simulink model "LOSR_old"  (R2022a)
settings: Solver=FixedStepDiscrete  StartTime=0.0  StopTime=0.04  FixedStep=0.04  RelTol=1e-3
PreLoadFcn:
  | listing = dir;
  | if (contains([listing .name], 'AGR')) && (contains([listing .name], 'MAP'))
  |     addpath('./AGR', './MAP');
  |     addpath( genpath('./MAP') );
  | elseif (contains([listing .name], 'LOSR.slx'))
  |     addpath('../AGR', '../MAP');
  |     addpath( genpath('../MAP') );
  | else
  | 
  | end
  | 
  | load('BusStructureLOSR.mat');
InitFcn:
  | listing = dir;
  | if (contains([listing .name], 'AGR')) && (contains([listing .name], 'MAP'))
  |     addpath('./AGR', './MAP');
  |     addpath( genpath('./MAP') );
  | elseif (contains([listing .name], 'LOSR.slx'))
  |     addpath('../AGR', '../MAP');
  |     addpath( genpath('../MAP') );
  | else
  | 
  | end
  | 
  | load('BusStructureLOSR.mat');
StartFcn:
  | listing = dir;
  | if (contains([listing .name], 'AGR')) && (contains([listing .name], 'MAP'))
  |     addpath('./AGR', './MAP');
  |     addpath( genpath('./MAP') );
  | elseif (contains([listing .name], 'LOSR.slx'))
  |     addpath('../AGR', '../MAP');
  |     addpath( genpath('../MAP') );
  | else
  | 
  | end
  | 
  | load('BusStructureLOSR.mat');
undefined symbols (not defined in the file): b2NED, delLLH, heading, llh, losECEF, losGeod, LOSRDataTagWrap, LOSRDataValid, LOSRDirectionCosineX, LOSRDirectionCosineY, LOSRDirectionCosineZ, LOSRSelected, LOSRSelectedWraparound, LOSRTargetElevation, LOSRTargetLatitude, LOSRTargetLongitude, LOSRTargetRangeEast, LOSRTargetRangeNorth, LOSRTargetRangeVertical, ne, ned2ECEF, pECEF_ref, pitch, roll, testLLH, testLLH2, testTerrainHeight
settings Model: Creator=ASCL  LastModifiedBy=ASCL
settings SolverCC: AlgebraicLoopSolver=TrustRegion
settings DataIOCC: SaveOutput=off  SignalLogging=off  DSMLogging=off  SaveTime=off  ReturnWorkspaceOutputs=off
settings OptimizationCC: DefaultParameterBehavior=Inlined  UseDivisionForNetSlopeComputation=on  GainParamInheritBuiltInType=on  UseFloatMulNetSlope=on  InlineInvariantSignals=on  BufferReuse=off  ExpressionFolding=off  PassReuseOutputArgsAs=Individual arguments  ZeroExternalMemoryAtStartup=off  ZeroInternalMemoryAtStartup=off  EfficientMapNaN2IntZero=off  LifeSpan=1  OptimizeBlockOrder=speed  DifferentSizesBufferReuse=on  EfficientTunableParamExpr=on
settings DebuggingCC: ParameterTunabilityLossMsg=error  UnconnectedInputMsg=warning  UnconnectedOutputMsg=warning  UnconnectedLineMsg=warning  SFMachineParentedDataDiag=warning  ArithmeticOperatorsInVariantConditions=warning
settings HardwareCC: ProdBitPerPointer=32  ProdBitPerSizeT=32  ProdBitPerPtrDiffT=32  ProdLargestAtomicInteger=Long  ProdLargestAtomicFloat=Double  ProdEndianess=BigEndian  ProdWordSize=32  ProdLongLongMode=on  ProdHWDeviceType=Freescale->MPC83xx
settings ModelReferenceCC: ModelReferenceNumInstancesAllowed=Single
settings SFSimCC: SimUserLibraries=MAPd.lib WS2_32.lib  SimUseLocalCustomCode=off  MATLABDynamicMemAlloc=off  CustomCodeUndefinedFunction=UseInterfaceOnly
settings SFSimCC: SimCustomHeaderCode=|
  | #include "MAP.h"
  | #include "DVOF.h"
  | #include "MAPDATA.h"
  | #include "userDefined.h"
settings SFSimCC: SimUserSources=|
  | MAP.c
  | DVOF.c
  | userDefined.c
settings RTWCC: SystemTargetFile=ert.tlc  TemplateMakefile=ert_default_tmf  GenerateReport=on  RTWUseLocalCustomCode=off  RTWUseSimCustomCode=on  CustomLibrary=MAPd.lib WS2_32.lib  IncludeHyperlinkInReport=on  LaunchReport=on  GenerateTraceInfo=on  GenerateTraceReport=on  GenerateTraceReportSl=on  GenerateTraceReportSf=on  GenerateTraceReportEml=on  GenerateCodeMetricsReport=on
settings RTWCC: CustomHeaderCode=|
  | #include "MAP.h"
  | #include "DVOF.h"
  | #include "MAPDATA.h"
  | #include "userDefined.h"
settings RTWCC: CustomSource=|
  | MAP.c
  | DVOF.c
  | userDefined.c
settings CodeAppCC: ForceParamTrailComments=on  IgnoreCustomStorageClasses=off  OperatorAnnotations=on  SimulinkDataObjDesc=on  SFDataObjDesc=on  InsertBlockDesc=on  EnableCustomComments=on
settings ERTTargetCC: TargetLangStandard=C99 (ISO)  UtilityFuncGeneration=Shared location  GenerateSampleERTMain=on  IncludeMdlTerminateFcn=off  CombineSignalStateStructs=on  SuppressErrorStatus=on  SupportAbsoluteTime=off  SupportComplex=off  InlinedParameterPlacement=NonHierarchical  ERTCustomFileTemplate=example_file_process.tlc  ERTFilePackagingFormat=CompactWithDataFile  EnableSignedLeftShifts=off  EnableSignedRightShifts=off

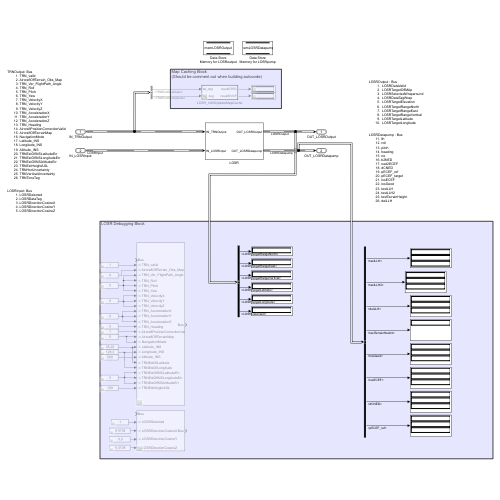
[thumbnail: Simulink's stored preview of the top-level diagram]
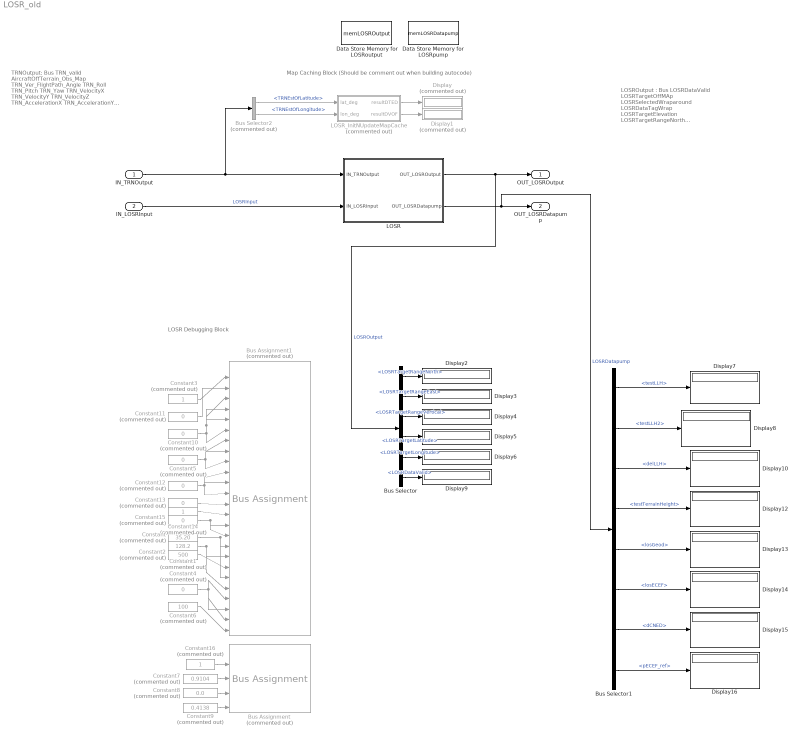
== system LOSR_old ==
  note: LOSR Debugging Block
  note: TRNOutput: Bus
      | TRN_valid
      | AircraftOffTerrain_Obs_Map
      | TRN_Ver_FlightPath_Angle
      | TRN_Roll
      | TRN_Pitch
      | TRN_Yaw
      | TRN_VelocityX
      | TRN_VelocityY
      | TRN_VelocityZ
      | TRN_AccelerationX
      | TRN_AccelerationY
      | TRN_AccelerationZ
      | TRN_Heading
      | AircraftPositionCorrectionValid
      | AircraftOffTerrainMap
      | NavigationMode
      | Latitude_INS
      | Longitude_INS
      | Altitude_INS
      | TRNEstOfINSLatitudeErr
      | TRNEstOfINSLongitudeErr
      | TRNEstOfINSAltitudeErr
      | TRNEstHeightAGL
      | TRNHorUncertainty
      | TRNVerticalUncertainty
      | TRNTimeTag
      |
      | LOSRInput: Bus
      | LOSRSelected
      | LOSRDataTag
      | LOSRDirectionCosineX
      | LOSRDirectionCosineY
      | LOSRDirectionCosineZ
  note: LOSROutput : Bus
      | LOSRDataValid
      | LOSRTargetOffMAp
      | LOSRSelectedWraparound
      | LOSRDataTagWrap
      | LOSRTargetElevation
      | LOSRTargetRangeNorth
      | LOSRTargetRangeEast
      | LOSRTargetRangeVertical
      | LOSRTargetLatitude
      | LOSRTargetLongitude
      |
      | LOSRDatapump : Bus
      | 11. llh
      | 12. roll
      | 13. pitch
      | 14. heading
      | 15. ne
      | 16. b2NED
      | 17. ned2ECEF
      | 18. dCNED
      | 19. pECEF_ref
      | 20. pECEF_target
      | 21. losECEF
      | 22. losGeod
      | 23. testLLH
      | 24. testLLH2
      | 25. testTerrainHeight
      | 26. delLLH
  note: Map Caching Block
      | (Should be comment out when building autocode)
  IN_TRNOutput : Inport  OutDataTypeStr=Bus: TRNOutput  BusOutputAsStruct=on
  IN_LOSRInput : Inport  Port=2  OutDataTypeStr=Bus: LOSRInput  BusOutputAsStruct=on
  Bus Assignment : BusAssignment  Commented=on  AssignedSignals=LOSRSelected,LOSRDirectionCosineX,LOSRDirectionCosineY,LOSRDirectionCosineZ
  Bus Assignment1 : BusAssignment  Commented=on  AssignedSignals=TRN_valid,AircraftOffTerrain_Obs_Map,TRN_Ver_FlightPath_Angle,TRN_Roll,TRN_Pitch,TRN_Yaw,TRN_VelocityX,TRN_VelocityY,TRN_VelocityZ,TRN_AccelerationX,TRN_AccelerationY,TRN_AccelerationZ,TRN_Heading,AircraftPositionCorrectionValid,AircraftOffTerrainMap,NavigationMode,Latitude_INS,Longitude_INS,Altitude_INS,TRNEstOfLatitude,TRNEstOfLongitude,TRNEstOfINSLatitudeErr,TRNEstOfINSLongitudeErr,TRNEstOfINSAltitudeErr,TRNEstHeightAGL
  Bus Selector : BusSelector  OutputSignals=LOSRTargetRangeNorth,LOSRTargetRangeEast,LOSRTargetRangeVertical,LOSRTargetLatitude,LOSRTargetLongitude,LOSRDataValid
  Bus Selector1 : BusSelector  OutputSignals=testLLH,testLLH2,delLLH,testTerrainHeight,losGeod,losECEF,dCNED,pECEF_ref
  Bus Selector2 : BusSelector  Commented=on  OutputSignals=TRNEstOfLatitude,TRNEstOfLongitude
  Constant : Constant  Commented=on  Value=35.20
  Constant1 : Constant  Commented=on  Value=128.2
  Constant{4..5,10,12..13} (5 alike) : Constant  Commented=on  Value=0
  Constant11 : Constant  Commented=on  Value=0  OutDataTypeStr=boolean
  Constant14 : Constant  Commented=on  OutDataTypeStr=boolean
  Constant15 : Constant  Commented=on  Value=0  OutDataTypeStr=boolean
  Constant16 : Constant  Commented=on  OutDataTypeStr=boolean
  Constant2 : Constant  Commented=on  Value=500
  Constant3 : Constant  Commented=on  OutDataTypeStr=boolean
  Constant6 : Constant  Commented=on  Value=100  OutDataTypeStr=uint16
  Constant7 : Constant  Commented=on  Value=0.9104
  Constant8 : Constant  Commented=on  Value=0.0
  Constant9 : Constant  Commented=on  Value=0.4138
  Data Store Memory for LOSRoutput : DataStoreMemory  DataStoreName=memLOSROutput  ReadBeforeWriteMsg=warning  WriteAfterWriteMsg=warning  WriteAfterReadMsg=warning  VectorParams1D=off  ShowAdditionalParam=off  OutDataTypeStr=Bus: LOSROutput
  Data Store Memory for LOSRpump : DataStoreMemory  DataStoreName=memLOSRDatapump  ReadBeforeWriteMsg=warning  WriteAfterWriteMsg=warning  WriteAfterReadMsg=warning  VectorParams1D=off  ShowAdditionalParam=off  OutDataTypeStr=Bus: LOSRDatapump
  Display : Display  Commented=on
  Display1 : Display  Commented=on
  Display{2..10,12..16} (14 alike) : Display
  LOSR : Subsystem
      mask init:
      | % latGPS = double(0);
      | % lonGPS = double(0);
      | % altGPS = double(0);
      | % velEGPS = double(0);
      | % velNGPS = double(0);
      | % velUGPS = double(0);
      | % notValidGPS = boolean(0);
      | % notAvaildINS = boolean(0);
      | % velUINS = double(0);
      | % velVINS = double(0);
      | % velWINS = double(0);
      | % rollINS = double(0);
      | % pitchINS = double(0);
      | % hgdINS = double(0);
      | % accXINS = double(0);
      | % accYINS = double(0);
      | % accZINS = double(0);
      | % activated = boolean(0);
      | % reactionT = uint16(0);
      | % pullUpG = uint16(0);
      | % rollRate = uint16(0);
      | % gOnsetRate = uint16(0);
      | % maxGamma = uint16(0);
      | % setWarnH = double(0);
      | % obsWarningTime = uint16(1);
      | % wiresWarningTime = uint16(1);
      | % latErrOfINS = double(0);
      | % lonErrOfINS = double(0);
      | % altErrorofINS = uint16(0);
      | % heightEstOfTRN = uint16(0);
      | % horUncertaintyOfTRN = double(0);
      | % verUncertaintyOfTRN = double(0);
  LOSR_InitNUpdateMapCache : Subsystem  Commented=on  TreatAsAtomicUnit=on
  OUT_LOSROutput : Outport  OutDataTypeStr=Bus: LOSROutput  VectorParamsAs1DForOutWhenUnconnected=off  BusOutputAsStruct=on
  OUT_LOSRDatapump : Outport  Port=2  OutDataTypeStr=Bus: LOSRDatapump  VectorParamsAs1DForOutWhenUnconnected=off  BusOutputAsStruct=on
  wires:
  LOSR/2(OUT_LOSRDatapump) -> Bus Selector1/1, OUT_LOSRDatapump/1  "LOSRDatapump"
  LOSR/1(OUT_LOSROutput) -> Bus Selector/1, OUT_LOSROutput/1  "LOSROutput"
  LOSR_InitNUpdateMapCache/2(resultDVOF) -> Display1/1
  Bus Selector/1 -> Display2/1  "<LOSRTargetRangeNorth>"
  Bus Selector/5 -> Display6/1  "<LOSRTargetLongitude>"
  Bus Selector/4 -> Display5/1  "<LOSRTargetLatitude>"
  Bus Selector/3 -> Display4/1  "<LOSRTargetRangeVertical>"
  Bus Selector/2 -> Display3/1  "<LOSRTargetRangeEast>"
  Bus Selector1/1 -> Display7/1  "<testLLH>"
  Bus Selector1/2 -> Display8/1  "<testLLH2>"
  Bus Selector/6 -> Display9/1  "<LOSRDataValid>"
  Bus Selector1/3 -> Display10/1  "<delLLH>"
  Bus Selector1/4 -> Display12/1  "<testTerrainHeight>"
  Bus Selector1/5 -> Display13/1  "<losGeod>"
  Bus Selector1/6 -> Display14/1  "<losECEF>"
  Bus Selector1/7 -> Display15/1  "<dCNED>"
  Bus Selector1/8 -> Display16/1  "<pECEF_ref>"
  LOSR_InitNUpdateMapCache/1(resultDTED) -> Display/1
  Constant9/1 -> Bus Assignment/5
  Constant7/1 -> Bus Assignment/3
  Constant8/1 -> Bus Assignment/4
  Constant1/1 -> Bus Assignment1/22, Bus Assignment1/19
  Constant/1 -> Bus Assignment1/21, Bus Assignment1/18
  Constant2/1 -> Bus Assignment1/20
  Constant4/1 -> Bus Assignment1/23, Bus Assignment1/25, Bus Assignment1/24
  Constant5/1 -> Bus Assignment1/10, Bus Assignment1/8, Bus Assignment1/9
  Constant10/1 -> Bus Assignment1/7, Bus Assignment1/4, Bus Assignment1/5, Bus Assignment1/6
  Constant3/1 -> Bus Assignment1/2
  Constant11/1 -> Bus Assignment1/3
  Constant12/1 -> Bus Assignment1/13, Bus Assignment1/11, Bus Assignment1/12
  Constant13/1 -> Bus Assignment1/14
  Constant14/1 -> Bus Assignment1/15
  Constant15/1 -> Bus Assignment1/17, Bus Assignment1/16
  Constant6/1 -> Bus Assignment1/26
  Bus Selector2/1 -> LOSR_InitNUpdateMapCache/1(lat_deg)  "<TRNEstOfLatitude>"
  Bus Selector2/2 -> LOSR_InitNUpdateMapCache/2(lon_deg)  "<TRNEstOfLongitude>"
  Constant16/1 -> Bus Assignment/2
  IN_TRNOutput/1 -> Bus Selector2/1, LOSR/1(IN_TRNOutput)
  IN_LOSRInput/1 -> LOSR/2(IN_LOSRInput)  "LOSRInput"

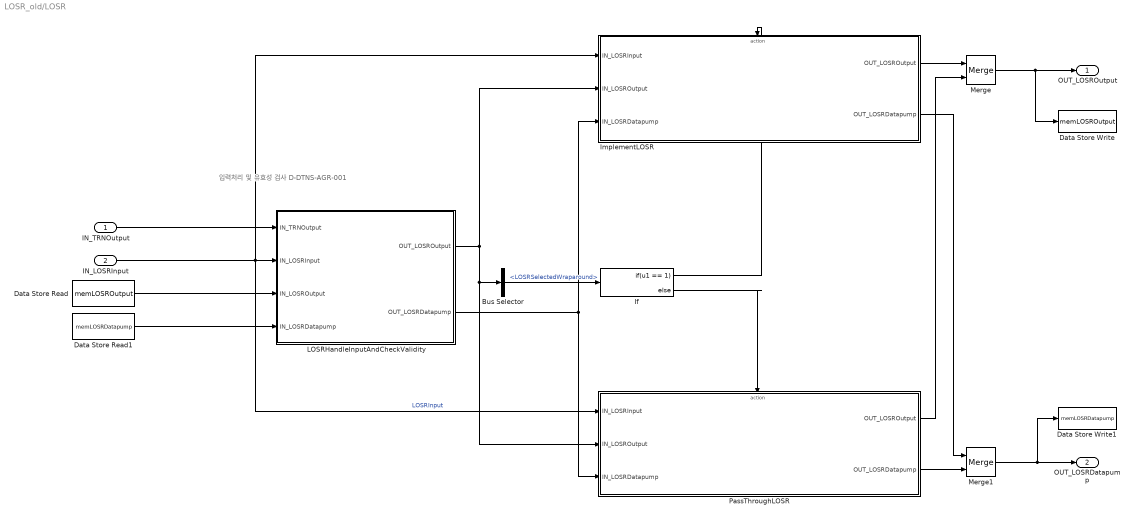
== system LOSR_old/LOSR ==
  note: 입력처리 및 유효성 검사 D-DTNS-AGR-001
  IN_TRNOutput : Inport  OutDataTypeStr=Bus: TRNOutput
  IN_LOSRInput : Inport  Port=2  OutDataTypeStr=Bus: LOSRInput
  Bus Selector : BusSelector  OutputSignals=LOSRSelectedWraparound
  Data Store Read : DataStoreRead  DataStoreName=memLOSROutput  IndexOptions=Index vector (dialog)  Indices=1  OutputSizes=1
  Data Store Read1 : DataStoreRead  DataStoreName=memLOSRDatapump  IndexOptions=Index vector (dialog)  Indices=1  OutputSizes=1
  Data Store Write : DataStoreWrite  DataStoreName=memLOSROutput  IndexOptions=Index vector (dialog)  Indices=1  OutputSizes=1
  Data Store Write1 : DataStoreWrite  DataStoreName=memLOSRDatapump  IndexOptions=Index vector (dialog)  Indices=1  OutputSizes=1
  If : If  IfExpression=u1 == 1
  ImplementLOSR : Subsystem  TreatAsAtomicUnit=on
      settings: RTWSystemCode=Nonreusable function  RTWFcnNameOpts=Use subsystem name
  LOSRHandleInputAndCheckValidity : Subsystem  TreatAsAtomicUnit=on
      settings: RTWSystemCode=Nonreusable function  RTWFcnNameOpts=Use subsystem name
  Merge : Merge
  Merge1 : Merge
  PassThroughLOSR : Subsystem  TreatAsAtomicUnit=on
      settings: RTWSystemCode=Nonreusable function  RTWFcnNameOpts=Use subsystem name
  OUT_LOSROutput : Outport  OutDataTypeStr=Bus: LOSROutput  VectorParamsAs1DForOutWhenUnconnected=off
  OUT_LOSRDatapump : Outport  Port=2  OutDataTypeStr=Bus: LOSRDatapump  VectorParamsAs1DForOutWhenUnconnected=off
  wires:
  IN_LOSRInput/1 -> ImplementLOSR/1(IN_LOSRInput), PassThroughLOSR/1(IN_LOSRInput), LOSRHandleInputAndCheckValidity/2(IN_LOSRInput)  "LOSRInput"
  LOSRHandleInputAndCheckValidity/1(OUT_LOSROutput) -> ImplementLOSR/2(IN_LOSROutput), Bus Selector/1, PassThroughLOSR/2(IN_LOSROutput)
  Bus Selector/1 -> If/1  "<LOSRSelectedWraparound>"
  If/1 -> ImplementLOSR/Action
  LOSRHandleInputAndCheckValidity/2(OUT_LOSRDatapump) -> ImplementLOSR/3(IN_LOSRDatapump), PassThroughLOSR/3(IN_LOSRDatapump)
  ImplementLOSR/1(OUT_LOSROutput) -> Merge/1
  PassThroughLOSR/2(OUT_LOSRDatapump) -> Merge1/2
  ImplementLOSR/2(OUT_LOSRDatapump) -> Merge1/1
  PassThroughLOSR/1(OUT_LOSROutput) -> Merge/2
  Merge/1 -> Data Store Write/1, OUT_LOSROutput/1
  Merge1/1 -> Data Store Write1/1, OUT_LOSRDatapump/1
  If/2 -> PassThroughLOSR/Action
  IN_TRNOutput/1 -> LOSRHandleInputAndCheckValidity/1(IN_TRNOutput)
  Data Store Read/1 -> LOSRHandleInputAndCheckValidity/3(IN_LOSROutput)
  Data Store Read1/1 -> LOSRHandleInputAndCheckValidity/4(IN_LOSRDatapump)

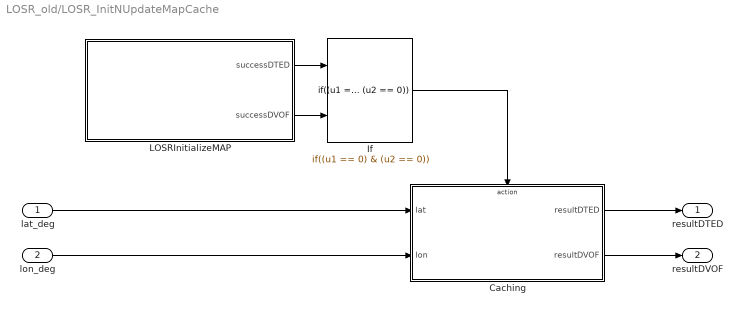
== system LOSR_old/LOSR_InitNUpdateMapCache ==
  lat_deg : Inport
  lon_deg : Inport  Port=2
  Caching : Subsystem  TreatAsAtomicUnit=on
  If : If  NumInputs=2  IfExpression=(u1 == 0) & (u2 == 0)  ShowElse=off
  LOSRInitializeMAP : MATLAB Function  TreatAsAtomicUnit=on
  resultDTED : Outport  VectorParamsAs1DForOutWhenUnconnected=off
  resultDVOF : Outport  Port=2  VectorParamsAs1DForOutWhenUnconnected=off
  wires:
  lon_deg/1 -> Caching/2(lon)
  Caching/1(resultDTED) -> resultDTED/1
  LOSRInitializeMAP/1(successDTED) -> If/1
  lat_deg/1 -> Caching/1(lat)
  Caching/2(resultDVOF) -> resultDVOF/1
  LOSRInitializeMAP/2(successDVOF) -> If/2
  If/1 -> Caching/Action

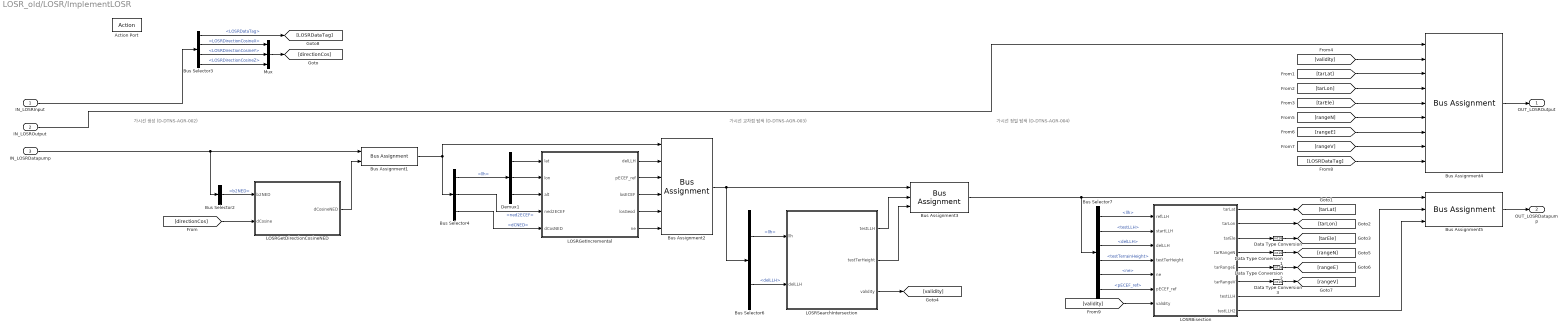
== system LOSR_old/LOSR/ImplementLOSR ==
  note: 가시선 생성 (D-DTNS-AGR-002)
  note: 가시선 교차점 탐색 (D-DTNS-AGR-003)
  note: 가시선 정밀 탐색 (D-DTNS-AGR-004)
  IN_LOSRInput : Inport  OutDataTypeStr=Bus: LOSRInput
  IN_LOSROutput : Inport  Port=2  OutDataTypeStr=Bus: LOSROutput
  IN_LOSRDatapump : Inport  Port=3  OutDataTypeStr=Bus: LOSRDatapump
  Action Port : ActionPort  ActionPortLabel=if(u1 == 1)
  Bus Assignment1 : BusAssignment  AssignedSignals=dCNED
  Bus Assignment2 : BusAssignment  AssignedSignals=delLLH,pECEF_ref,losECEF,losGeod,ne
  Bus Assignment3 : BusAssignment  AssignedSignals=testLLH,testTerrainHeight
  Bus Assignment4 : BusAssignment  AssignedSignals=LOSRDataValid,LOSRTargetLatitude,LOSRTargetLongitude,LOSRTargetElevation,LOSRTargetRangeNorth,LOSRTargetRangeEast,LOSRTargetRangeVertical,LOSRDataTagWrap
  Bus Assignment5 : BusAssignment  AssignedSignals=testLLH,testLLH2
  Bus Selector2 : BusSelector  OutputSignals=b2NED
  Bus Selector3 : BusSelector  OutputSignals=LOSRDataTag,LOSRDirectionCosineX,LOSRDirectionCosineY,LOSRDirectionCosineZ
  Bus Selector4 : BusSelector  OutputSignals=llh,ned2ECEF,dCNED
  Bus Selector6 : BusSelector  OutputSignals=llh,delLLH
  Bus Selector7 : BusSelector  OutputSignals=llh,testLLH,delLLH,testTerrainHeight,ne,pECEF_ref
  Data Type Conversion{,1..3} (4 alike) : DataTypeConversion  OutDataTypeStr=int16  SaturateOnIntegerOverflow=off  RndMeth=Floor
  Demux1 : Demux  Outputs=3
  LOSRBisection : MATLAB Function  TreatAsAtomicUnit=on
      settings: RTWSystemCode=Nonreusable function  RTWFcnNameOpts=Use subsystem name
  LOSRGetDirectionCosineNED : MATLAB Function  TreatAsAtomicUnit=on
      settings: RTWSystemCode=Nonreusable function  RTWFcnNameOpts=Use subsystem name
  LOSRGetIncremental : MATLAB Function  TreatAsAtomicUnit=on
      settings: RTWSystemCode=Nonreusable function  RTWFcnNameOpts=Use subsystem name
  LOSRSearchIntersection : MATLAB Function  TreatAsAtomicUnit=on
      settings: RTWSystemCode=Nonreusable function  RTWFcnNameOpts=Use subsystem name
  Mux : Mux  Inputs=3
  OUT_LOSROutput : Outport  OutDataTypeStr=Bus: LOSROutput  VectorParamsAs1DForOutWhenUnconnected=off
  OUT_LOSRDatapump : Outport  Port=2  OutDataTypeStr=Bus: LOSRDatapump  VectorParamsAs1DForOutWhenUnconnected=off
  wires:
  Bus Assignment3/1 -> Bus Assignment5/1, Bus Selector7/1
  LOSRSearchIntersection/3(validity) -> [validity]
  [tarLat] -> Bus Assignment4/3
  LOSRBisection/5(tarRangeE) -> Data Type Conversion2/1
  LOSRBisection/2(tarLon) -> [tarLon]
  Bus Selector7/6 -> LOSRBisection/6(pECEF_ref)  "<pECEF_ref>"
  LOSRSearchIntersection/1(testLLH) -> Bus Assignment3/2
  [rangeV] -> Bus Assignment4/8
  Bus Selector7/3 -> LOSRBisection/3(delLLH)  "<delLLH>"
  [directionCos] -> LOSRGetDirectionCosineNED/2(dCosine)
  [tarEle] -> Bus Assignment4/5
  Bus Selector6/2 -> LOSRSearchIntersection/2(delLLH)  "<delLLH>"
  Bus Selector4/3 -> LOSRGetIncremental/5(dCosNED)  "<dCNED>"
  LOSRGetIncremental/4(losGeod) -> Bus Assignment2/5
  LOSRGetIncremental/2(pECEF_ref) -> Bus Assignment2/3
  Demux1/3 -> LOSRGetIncremental/3(alt)
  Bus Assignment2/1 -> Bus Assignment3/1, Bus Selector6/1
  Bus Selector2/1 -> LOSRGetDirectionCosineNED/1(b2NED)  "<b2NED>"
  [tarLon] -> Bus Assignment4/4
  Bus Selector3/3 -> Mux/2  "<LOSRDirectionCosineY>"
  Bus Selector3/2 -> Mux/1  "<LOSRDirectionCosineX>"
  Bus Selector6/1 -> LOSRSearchIntersection/1(llh)  "<llh>"
  Bus Assignment1/1 -> Bus Selector4/1, Bus Assignment2/1
  Bus Selector4/1 -> Demux1/1  "<llh>"
  Bus Selector3/1 -> [LOSRDataTag]  "<LOSRDataTag>"
  Bus Selector4/2 -> LOSRGetIncremental/4(ned2ECEF)  "<ned2ECEF>"
  Bus Selector7/5 -> LOSRBisection/5(ne)  "<ne>"
  IN_LOSROutput/1 -> Bus Assignment4/1
  Bus Selector7/4 -> LOSRBisection/4(testTerHeight)  "<testTerrainHeight>"
  LOSRBisection/3(tarEle) -> Data Type Conversion/1
  [rangeN] -> Bus Assignment4/6
  LOSRBisection/1(tarLat) -> [tarLat]
  Data Type Conversion2/1 -> [rangeE]
  IN_LOSRDatapump/1 -> Bus Assignment1/1, Bus Selector2/1
  Bus Selector7/2 -> LOSRBisection/2(startLLH)  "<testLLH>"
  Data Type Conversion1/1 -> [rangeN]
  Mux/1 -> [directionCos]
  [rangeE] -> Bus Assignment4/7
  Data Type Conversion/1 -> [tarEle]
  LOSRBisection/7(testLLH) -> Bus Assignment5/2
  LOSRSearchIntersection/2(testTerHeight) -> Bus Assignment3/3
  LOSRBisection/4(tarRangeN) -> Data Type Conversion1/1
  Data Type Conversion3/1 -> [rangeV]
  LOSRGetIncremental/1(delLLH) -> Bus Assignment2/2
  LOSRBisection/8(testLLH2) -> Bus Assignment5/3
  LOSRBisection/6(tarRangeV) -> Data Type Conversion3/1
  LOSRGetIncremental/3(losECEF) -> Bus Assignment2/4
  LOSRGetDirectionCosineNED/1(dCosineNED) -> Bus Assignment1/2
  [validity] -> Bus Assignment4/2
  IN_LOSRInput/1 -> Bus Selector3/1
  Bus Assignment4/1 -> OUT_LOSROutput/1
  Bus Assignment5/1 -> OUT_LOSRDatapump/1
  Bus Selector3/4 -> Mux/3  "<LOSRDirectionCosineZ>"
  [LOSRDataTag] -> Bus Assignment4/9
  Bus Selector7/1 -> LOSRBisection/1(refLLH)  "<llh>"
  Demux1/1 -> LOSRGetIncremental/1(lat)
  Demux1/2 -> LOSRGetIncremental/2(lon)
  LOSRGetIncremental/5(ne) -> Bus Assignment2/6
  [validity] -> LOSRBisection/7(validity)

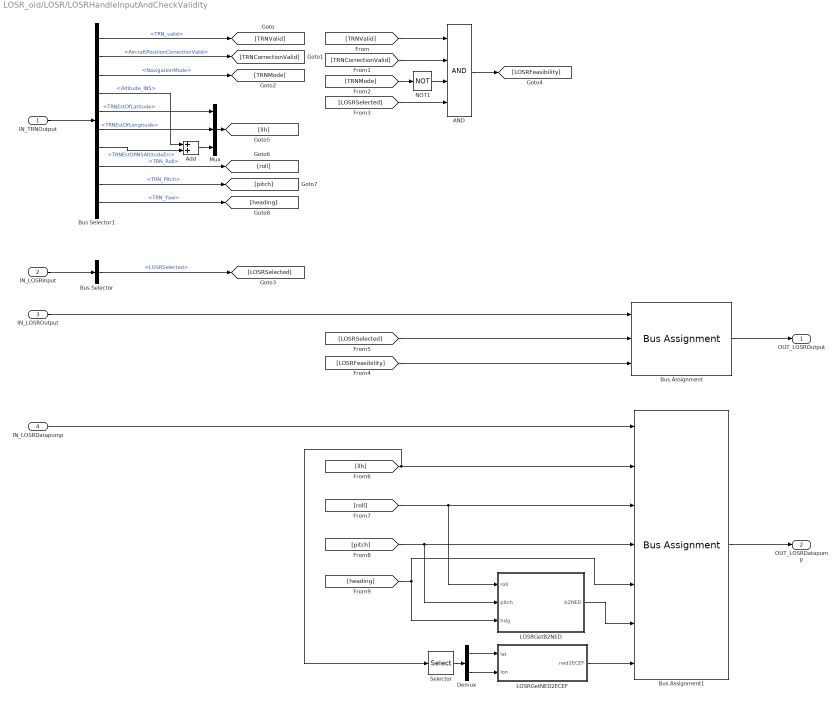
== system LOSR_old/LOSR/LOSRHandleInputAndCheckValidity ==
  IN_TRNOutput : Inport  OutDataTypeStr=Bus: TRNOutput
  IN_LOSRInput : Inport  Port=2  OutDataTypeStr=Bus: LOSRInput
  IN_LOSROutput : Inport  Port=3  OutDataTypeStr=Bus: LOSROutput
  IN_LOSRDatapump : Inport  Port=4  OutDataTypeStr=Bus: LOSRDatapump
  AND : Logic  Inputs=4  AllPortsSameDT=off  OutDataTypeStr=boolean
  Add : Sum
  Bus Assignment : BusAssignment  AssignedSignals=LOSRSelectedWraparound,LOSRDataValid
  Bus Assignment1 : BusAssignment  AssignedSignals=llh,roll,pitch,heading,b2NED,ned2ECEF
  Bus Selector : BusSelector  OutputSignals=LOSRSelected
  Bus Selector1 : BusSelector  OutputSignals=TRN_valid,AircraftPositionCorrectionValid,NavigationMode,Altitude_INS,TRNEstOfLatitude,TRNEstOfLongitude,TRNEstOfINSAltitudeErr,TRN_Roll,TRN_Pitch,TRN_Yaw
  Demux : Demux  Outputs=2
  LOSRGetB2NED : MATLAB Function  TreatAsAtomicUnit=on
  LOSRGetNED2ECEF : MATLAB Function  TreatAsAtomicUnit=on
  Mux : Mux  Inputs=3
  NOT1 : Logic  Operator=NOT  IconShape=distinctive  AllPortsSameDT=off  OutDataTypeStr=boolean
  Selector : Selector  InputPortWidth=3  IndexOptions=Index vector (dialog)  Indices=[1 2]  OutputSizes=1
  OUT_LOSROutput : Outport  OutDataTypeStr=Bus: LOSROutput  VectorParamsAs1DForOutWhenUnconnected=off
  OUT_LOSRDatapump : Outport  Port=2  OutDataTypeStr=Bus: LOSRDatapump  VectorParamsAs1DForOutWhenUnconnected=off
  wires:
  IN_LOSRDatapump/1 -> Bus Assignment1/1
  IN_LOSROutput/1 -> Bus Assignment/1
  Bus Assignment/1 -> OUT_LOSROutput/1
  IN_TRNOutput/1 -> Bus Selector1/1
  Bus Selector1/1 -> [TRNValid]  "<TRN_valid>"
  Bus Selector1/2 -> [TRNCorrectionValid]  "<AircraftPositionCorrectionValid>"
  Bus Selector1/3 -> [TRNMode]  "<NavigationMode>"
  IN_LOSRInput/1 -> Bus Selector/1
  Bus Selector/1 -> [LOSRSelected]  "<LOSRSelected>"
  [TRNValid] -> AND/1
  [TRNCorrectionValid] -> AND/2
  [TRNMode] -> NOT1/1
  [LOSRSelected] -> AND/4
  AND/1 -> [LOSRFeasibility]
  [LOSRSelected] -> Bus Assignment/2
  [LOSRFeasibility] -> Bus Assignment/3
  Bus Assignment1/1 -> OUT_LOSRDatapump/1
  LOSRGetNED2ECEF/1(ned2ECEF) -> Bus Assignment1/7
  LOSRGetB2NED/1(b2NED) -> Bus Assignment1/6
  Bus Selector1/4 -> Add/1  "<Altitude_INS>"
  Bus Selector1/5 -> Mux/1  "<TRNEstOfLatitude>"
  Bus Selector1/6 -> Mux/2  "<TRNEstOfLongitude>"
  Add/1 -> Mux/3
  Bus Selector1/7 -> Add/2  "<TRNEstOfINSAltitudeErr>"
  Mux/1 -> [llh]
  Bus Selector1/10 -> [heading]  "<TRN_Yaw>"
  Bus Selector1/9 -> [pitch]  "<TRN_Pitch>"
  Bus Selector1/8 -> [roll]  "<TRN_Roll>"
  [llh] -> Bus Assignment1/2, Selector/1
  Selector/1 -> Demux/1
  Demux/2 -> LOSRGetNED2ECEF/2(lon)
  Demux/1 -> LOSRGetNED2ECEF/1(lat)
  [roll] -> Bus Assignment1/3, LOSRGetB2NED/1(roll)
  [pitch] -> Bus Assignment1/4, LOSRGetB2NED/2(pitch)
  [heading] -> Bus Assignment1/5, LOSRGetB2NED/3(hdg)
  NOT1/1 -> AND/3

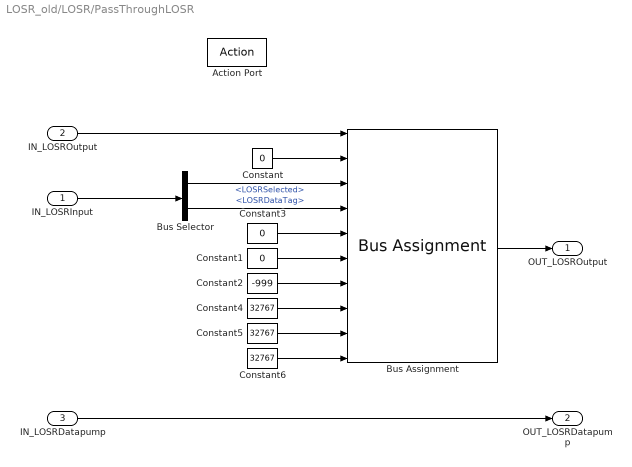
== system LOSR_old/LOSR/PassThroughLOSR ==
  IN_LOSRInput : Inport  OutDataTypeStr=Bus: LOSRInput
  IN_LOSROutput : Inport  Port=2  OutDataTypeStr=Bus: LOSROutput
  IN_LOSRDatapump : Inport  Port=3  OutDataTypeStr=Bus: LOSRDatapump
  Action Port : ActionPort  ActionPortLabel=else
  Bus Assignment : BusAssignment  AssignedSignals=LOSRDataValid,LOSRSelectedWraparound,LOSRDataTagWrap,LOSRTargetLatitude,LOSRTargetLongitude,LOSRTargetElevation,LOSRTargetRangeNorth,LOSRTargetRangeEast,LOSRTargetRangeVertical
  Bus Selector : BusSelector  OutputSignals=LOSRSelected,LOSRDataTag
  Constant : Constant  Value=0  OutDataTypeStr=boolean
  Constant1 : Constant  Value=0
  Constant2 : Constant  Value=-999  OutDataTypeStr=int16
  Constant3 : Constant  Value=0
  Constant4 : Constant  Value=32767  OutDataTypeStr=int16
  Constant5 : Constant  Value=32767  OutDataTypeStr=int16
  Constant6 : Constant  Value=32767  OutDataTypeStr=int16
  OUT_LOSROutput : Outport  OutDataTypeStr=Bus: LOSROutput  VectorParamsAs1DForOutWhenUnconnected=off
  OUT_LOSRDatapump : Outport  Port=2  OutDataTypeStr=Bus: LOSRDatapump  VectorParamsAs1DForOutWhenUnconnected=off
  wires:
  IN_LOSROutput/1 -> Bus Assignment/1
  IN_LOSRDatapump/1 -> OUT_LOSRDatapump/1
  IN_LOSRInput/1 -> Bus Selector/1
  Constant/1 -> Bus Assignment/2
  Bus Assignment/1 -> OUT_LOSROutput/1
  Bus Selector/1 -> Bus Assignment/3  "<LOSRSelected>"
  Bus Selector/2 -> Bus Assignment/4  "<LOSRDataTag>"
  Constant2/1 -> Bus Assignment/7
  Constant1/1 -> Bus Assignment/6
  Constant3/1 -> Bus Assignment/5
  Constant4/1 -> Bus Assignment/8
  Constant5/1 -> Bus Assignment/9
  Constant6/1 -> Bus Assignment/10

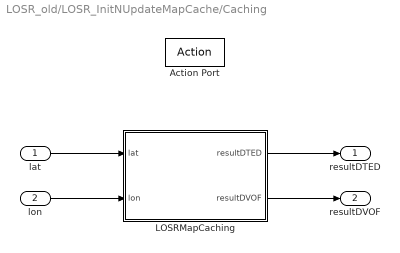
== system LOSR_old/LOSR_InitNUpdateMapCache/Caching ==
  lat : Inport
  lon : Inport  Port=2
  Action Port : ActionPort  ActionPortLabel=if((u1 == 0) & (u2 == 0))
  LOSRMapCaching : MATLAB Function  TreatAsAtomicUnit=on
  resultDTED : Outport  VectorParamsAs1DForOutWhenUnconnected=off
  resultDVOF : Outport  Port=2  VectorParamsAs1DForOutWhenUnconnected=off
  wires:
  LOSRMapCaching/1(resultDTED) -> resultDTED/1
  lat/1 -> LOSRMapCaching/1(lat)
  lon/1 -> LOSRMapCaching/2(lon)
  LOSRMapCaching/2(resultDVOF) -> resultDVOF/1

== matlab function LOSR_old/LOSR/LOSRHandleInputAndCheckValidity/LOSRGetNED2ECEF ==
  data: lat input; ned2ECEF output; lon input
function ned2ECEF = LOSRGetNED2ECEF(lat, lon)
%LOSRGetNED2ECEF Compute transformation matrix from local NED to ECEF frame
% Input
% lat       : Current aircraft latitude [deg]
% lon       : Current aircraft longitude [deg]
% Output
% ned2ECEF  : Rotation matrix in single 1D array form
% *Note : (ECEF Vecotr) = (ned2ECEF) * (NED Vector) + (ECEF, Reference)

% Initialize
ned2ECEF = zeros(1,9);

% NED to ECEF Transformation Matrix
ned2ECEF(1,1) = -sind(lat)*cosd(lon);
ned2ECEF(1,2) = -sind(lon);
ned2ECEF(1,3) = -cosd(lat)*cosd(lon);

ned2ECEF(1,4) = -sind(lat)*sind(lon);
ned2ECEF(1,5) = cosd(lon);
ned2ECEF(1,6) = -cosd(lat)*sind(lon);

ned2ECEF(1,7) = cosd(lat);
ned2ECEF(1,8) = 0.0;
ned2ECEF(1,9) = -sind(lat);

end

== matlab function LOSR_old/LOSR/ImplementLOSR/LOSRGetDirectionCosineNED ==
  data: b2NED input; dCosineNED output; dCosine input
function dCosineNED = LOSRGetDirectionCosineNED(b2NED, dCosine)
%LOSRGetDirectionCosineNED
% Compute Direction Cosine in NED frame using Body to NED transformation
% Input
% b2NED     : Body to NED Transformation matrix in single 1D array form
% dCosine   : Direction Cosine X, Y, Z
% Output
% dCosineNED: Direction Cosine in North, East, Down

% Initialize
dCosineNED    = zeros(3,1);

dCosineNED(1) = b2NED(1)*dCosine(1) + b2NED(2)*dCosine(2) + b2NED(3)*dCosine(3);
dCosineNED(2) = b2NED(4)*dCosine(1) + b2NED(5)*dCosine(2) + b2NED(6)*dCosine(3);
dCosineNED(3) = b2NED(7)*dCosine(1) + b2NED(8)*dCosine(2) + b2NED(9)*dCosine(3);
end

== matlab function LOSR_old/LOSR/ImplementLOSR/LOSRGetIncremental ==
  data: lat input; lon input; delLLH output; alt input; ned2ECEF input; dCosNED input; pECEF_ref output; losECEF output; losGeod output; ne output
function [delLLH, pECEF_ref, losECEF, losGeod, ne] = LOSRGetIncremental(lat, lon, alt, ned2ECEF, dCosNED)
%LOSRGetIncremental
% Compute Direction Cosine in NED frame using Body to NED transformation
% Input
% lat       : Current aircraft latitude [deg]
% lon       : Current aircraft longitude [deg]
% alt       : Current aircraft altitude [m]
% dCosineNED: Direction Cosine in North, East, Down
% dCosine   : Direction Cosine X, Y, Z
% losiMaxSteps   : Maximum LOSI Alrogithm steps
% Output
% delLLH
% pECEF_ref
% losECEF
% losGeod
% ne        : Prime vertical radius of curvature

% Initialize Output
delLLH          = zeros(3,1);
pECEF_ref       = zeros(3,1);
losECEF         = zeros(3,1);
losGeod         = zeros(3,1);

% Define constants
R_Ea            = 6378137.0;        % Earth semi-major axis [m]
e               = 0.08181919;       % Earth eccentricity
LOSI_MAX_STEPS  = 640;

% Prime vertical radius of curvature
ne              = R_Ea / sqrt(1 - (e * sind(lat))^2 );
me              = R_Ea * (1 - e^2) / (1 - e^2*(sind(lat))^2)^(3/2);

% Define reference point in ECEF coordinates
pECEF_ref(1)    = (ne+alt) * cosd(lat) * cosd(lon);
pECEF_ref(2)    = (ne+alt) * cosd(lat) * sind(lon);
pECEF_ref(3)    = (ne * ( 1 - e^2 ) + alt) * sind(lat);

% LOS in ECEF 
losECEF(1)      = ned2ECEF(1)*dCosNED(1) + ned2ECEF(2)*dCosNED(2) + ned2ECEF(3)*dCosNED(3) + pECEF_ref(1);
losECEF(2)      = ned2ECEF(4)*dCosNED(1) + ned2ECEF(5)*dCosNED(2) + ned2ECEF(6)*dCosNED(3) + pECEF_ref(2);
losECEF(3)      = ned2ECEF(7)*dCosNED(1) + ned2ECEF(8)*dCosNED(2) + ned2ECEF(9)*dCosNED(3) + pECEF_ref(3);

% LOS in Geod
losGeod(1)      = dCosNED(1) / (me+alt) * 180/pi;
losGeod(2)      = dCosNED(2) / (ne+alt) / cosd(lat) * 180/pi;
losGeod(3)      = -dCosNED(3);

% LOS Length Control
delLLH          = losGeod * sqrt(20000^2+20000^2) / (LOSI_MAX_STEPS-1);
if norm(losECEF - pECEF_ref) > 0.1
    delECEF = (losECEF - pECEF_ref) / norm(losECEF - pECEF_ref) * 45;
else
    delECEF = zeros(3,1);
end
% scaler          = sqrt( losGeod(1)^2 + losGeod(2)^2 );
% delLLH          = losGeod / scaler * LOSR_TEST_INTER;
% % *Note : (ECEF Vecotr) = (ned2ECEF) * (NED Vector) + (ECEF, Reference)


end

== matlab function LOSR_old/LOSR/ImplementLOSR/LOSRSearchIntersection ==
  data: llh input; delLLH input; testLLH output; testTerHeight output; validity output
function [testLLH, testTerHeight, validity] = LOSRSearchIntersection(llh, delLLH)

% Initialize Variables
testLLH         = zeros(3,1);
tempTerHeight   = 0.0;
tempObsHeight   = 0.0;
testTerHeight   = 0.0;
validity        = true;
AMSLI           = 0;
AMSL            = 0;
index           = 0;
latOut          = 0.0;
lonOut          = 0.0;


% Define
LOSI_MAX_STEPS = 640;

% Searching LOS Intersection
for ii=0:(LOSI_MAX_STEPS-1)
    testLLH(1) = llh(1) + ii*delLLH(1);
    testLLH(2) = llh(2) + ii*delLLH(2);
    testLLH(3) = llh(3) + ii*delLLH(3);
    
    % Get Terrain Elevation
    tempTerHeight  = coder.ceval('GetElevation', testLLH(1), testLLH(2));
    
    % Get Obstacle Info
    index = coder.ceval('GetObstTotalCount');
    AMSL  = 0;
    if (index >= 0)
        for jj=0:index-1
            latOut = coder.ceval('GetObstacleInfo', testLLH(1), testLLH(2), jj, 1);
            lonOut = coder.ceval('GetObstacleInfo', testLLH(1), testLLH(2), jj, 2);
            dist=sqrt(((llh(1)-latOut)*pi/180*6378137)^2+((llh(2)-lonOut)*pi/180*6378137)^2);
            if (dist<50)
                AMSLI = coder.ceval('GetObstacleInfo', testLLH(1), testLLH(2), jj, 4);
                if (AMSLI>AMSL)
                    AMSL=AMSLI;
                end
            end
        end
    end
    tempObsHeight   = AMSL;
    
    % Get Highest Profile
    if ( tempTerHeight > tempObsHeight )
        testTerHeight = tempTerHeight;
    else
        testTerHeight = tempObsHeight;
    end
    
    if (testTerHeight >= testLLH(3))
        
        if ii==0
            % LOS Intersection is not possible
            validity = false;
            break;
        else
            % LOS Intersection exists
            validity = true;
            break;
        end
        
    else
        if (ii==LOSI_MAX_STEPS-1)
        % Max iteration is over without intersection found
        validity = false;
        end
        continue;
    end
    
end

end

== matlab function LOSR_old/LOSR/ImplementLOSR/LOSRBisection ==
  data: refLLH input; startLLH input; tarLat output; delLLH input; testTerHeight input; ne input; pECEF_ref input; tarLon output; tarEle output; tarRangeN output; tarRangeE output; tarRangeV output; testLLH output; testLLH2 output; validity input
function [tarLat, tarLon, tarEle, tarRangeN, tarRangeE, tarRangeV, testLLH, testLLH2]  = LOSRBisection(refLLH, startLLH, delLLH, testTerHeight, ne, pECEF_ref, validity)
% Initialize Output
tarLat      = 0.0;
tarLon      = 0.0;
tarEle      = 0.0;
tarRangeN   = 0.0;
tarRangeE   = 0.0;
tarRangeV   = 0.0;
testLLH     = zeros(3,1);
testLLH2    = zeros(3,1);
targetRange = zeros(3,1);
pECEF_target= zeros(3,1);
ecef2NED    = zeros(3,3);

% Constants
MAX_BISECTION   = 30;
TOL_BISECTION   = 0.5;

% Test Points
testLLH         = startLLH;
testLLH2        = startLLH - delLLH;

temp1= 0.0; temp2=0.0;

temp1 = coder.ceval('GetElevation', testLLH(1), testLLH(2));
temp2 = coder.ceval('GetElevation', testLLH2(1), testLLH2(2));
% fprintf("Terrain 1: %f, Terrain 2: %f \r\n", temp1, temp2);

if (validity == false)
    
    tarLat = 0;
    tarLon = 0;
    tarEle = -999;
    tarRangeN = 32767;
    tarRangeE = 32767;
    tarRangeV = 32767;
    
else
    for ii=0:(MAX_BISECTION -1)
        testTerHeight = coder.ceval('GetElevation', (testLLH(1) + testLLH2(1))/2, (testLLH(2) + testLLH2(2))/2 );

        if ( abs(testTerHeight - (testLLH(3)+testLLH2(3))/2) < TOL_BISECTION )
            break;
        end

%         fprintf('Current Index: %f \r\n', ii);
%         fprintf('testLLH: %f, %f, %f \r\n', testLLH(1), testLLH(2), testLLH(3));
%         fprintf('testLLH2: %f, %f, %f \r\n', testLLH2(1), testLLH2(2), testLLH2(3));

        if ( testTerHeight < (testLLH(3) + testLLH2(3))/2 )
            testLLH2(1)     = (testLLH(1) + testLLH2(1)) /2;
            testLLH2(2)     = (testLLH(2) + testLLH2(2)) /2;
            testLLH2(3)     = (testLLH(3) + testLLH2(3)) /2;
        else
            testLLH(1)      = (testLLH(1) + testLLH2(1)) /2;
            testLLH(2)      = (testLLH(2) + testLLH2(2)) /2;
            testLLH(3)      = (testLLH(3) + testLLH2(3)) /2;
        end

    end
    
    EARTH_ECCENTRICITY      = 0.08181919;

    tarLat           = (testLLH(1) + testLLH2(1)) /2;
    tarLon           = (testLLH(2) + testLLH2(2)) /2;
    tarEle           = (testLLH(3) + testLLH2(3)) /2;

    % Calculate Output
    pECEF_target(1)     = (ne + testTerHeight)*cosd(tarLat)*cosd(tarLon);
    pECEF_target(2)     = (ne + testTerHeight)*cosd(tarLat)*sind(tarLon);
    pECEF_target(3)     = (ne * (1 - EARTH_ECCENTRICITY^2) + testTerHeight) * sind(tarLat);

    ecef2NED    = [ -sind(refLLH(1)) * cosd(refLLH(2)), -sind(refLLH(1)) * sind(refLLH(2)), cosd(refLLH(1));
                    -sind(refLLH(2)),                   cosd(refLLH(2)),                    0;
                    -cosd(refLLH(1)) * cosd(refLLH(2)), -cosd(refLLH(1)) * sind(refLLH(2)), -sind(refLLH(1))];

    targetRange = ecef2NED * (pECEF_target - pECEF_ref);

    tarRangeN           = targetRange(1);
    tarRangeE           = targetRange(2);
    tarRangeV           = -targetRange(3);

end

end

== matlab function LOSR_old/LOSR_InitNUpdateMapCache/Caching/LOSRMapCaching ==
  data: resultDTED output; resultDVOF output; lat input; lon input
function [resultDTED, resultDVOF] = LOSRMapCaching(lat, lon)

resultDTED = int32(1);
resultDVOF = int32(1);

resultDVOF = coder.ceval('UpdateObstList', lat, lon);
resultDTED = coder.ceval('UpdateMapCache', lat, lon);

== matlab function LOSR_old/LOSR_InitNUpdateMapCache/LOSRInitializeMAP ==
  data: successDTED output; successDVOF output
function [successDTED, successDVOF] = LOSRInitializeMAP()

flagDTED = int32(1);
flagDVOF = int32(1);

pathDTED = 'C:\Users\ASCL\Documents\GitHub\DTNS\MAP\MAP_DB\';
pathDVOF = 'C:\Users\ASCL\Documents\GitHub\DTNS\MAP\DVOF\';

strLenDTED = int32(strlength(pathDTED));
strLenDVOF = int32(strlength(pathDVOF));

flagDTED = coder.ceval('InitialMap', pathDTED, strLenDTED );
flagDVOF = coder.ceval('InitDVOF', pathDVOF, strLenDVOF );

successDTED = flagDTED;
successDVOF = flagDVOF;

== matlab function LOSR_old/LOSR/LOSRHandleInputAndCheckValidity/LOSRGetB2NED ==
  data: roll input; b2NED output; pitch input; hdg input
function b2NED = LOSRGetB2NED(roll, pitch, hdg)
%LOSRGetNED2ECEF Compute transformation matrix from Body to local NED frame
% Input
% roll      : Current aircraft roll angle [deg]
% pitch     : Current aircraft pitch angle [deg]
% heading   : Current aircraft heading angle [deg]
% Output
% b2NED     : Transformation matrix in single 1D array form

% Initialize
b2NED = zeros(1,9);

b2NED(1,1)  = cosd(hdg) * cosd(pitch);
b2NED(1,2)  = -sind(hdg) * cosd(roll) + cosd(hdg) * sind(pitch) * sind(roll);
b2NED(1,3)  = sind(hdg) * sind(roll) + cosd(hdg) * sind(pitch) * cosd(roll);

b2NED(1,4)  = sind(hdg) * cosd(roll);
b2NED(1,5)  = cosd(hdg) * cosd(pitch) + sind(hdg) * sind(pitch) * sind(roll);
b2NED(1,6)  = -cosd(hdg) * sind(roll) + sind(hdg) * sind(pitch) * cosd(roll);

b2NED(1,7)  = -sind(pitch);
b2NED(1,8)  = cosd(pitch) * sind(roll);
b2NED(1,9)  = cosd(pitch) * cosd(roll);

end
